simulink model "fcs_mpc"  (Simulink 9.0)
settings: Solver=VariableStepAuto  StartTime=0.0  StopTime=120  RelTol=1e-3
values from neighbouring files (symbols this model uses):
  Bf = 10000    [parameters.m]
  Bw = 1.7    [parameters.m]
  c = 2.1e-8    (= 2.1e-08)    [parameters.m]
  F_OmegaI = [-0.0162184150400002, -0.00631156082725452, -0.00162300350054704; 0.0162184150400002, 0.00631156082725452, 0.00162300350054704; -1.91252880199500e-16, 0.0704545731974788, 0; 1.91252880199500e-16, -0.0704545731974788, 0; 0.00203835199999989, 0.0823409037568373, 0.0338642741053293; -0.00203835199999989, -0.0823409037568373, -0.0338642741053293; -0.000739879228098683, -0.0271199969505346, 0.003148463 ...(+73 chars)    [parameters.m]
  F_OmegaO = [1, 0, 0; -1, 0, 0; 0, 1, 0; 0, -1, 0; 0, 0, 1; 0, 0, -1]    [parameters.m]
  g_OmegaI = [0.00133150970594632; 0.00133150970594632; 0.00320850126341322; 0.00320850126341322; 0.00334621106108639; 0.00334621106108639; 0.00174333401990860; 0.00174333401990860]    [parameters.m]
  g_OmegaO = [0.1; 0.1; 0.046; 0.046; 0.2; 0.2]    [parameters.m]
  Hc = 9    [parameters.m]
  Hp = 23    [parameters.m]
  initial_theta = deg2rad(9)    [parameters.m]
  initial_x = 0    [parameters.m]
  initial_y = 0.05    [parameters.m]
  J = 50    [parameters.m]
  Jw = 5    [parameters.m]
  K = 1    [parameters.m]
  Kp = 20    [parameters.m]
  L = Lr + Lf    (= 1.58)    [parameters.m]
  Lf = 0.79    [parameters.m]
  Lr = 0.79    [parameters.m]
  Lw = 0.54    [parameters.m]
  M = 250    [parameters.m]
  omega_f = 0.3253    [parameters.m]
  phi_max = 0.61    [parameters.m]
  R = 0.29    [parameters.m]
  r = 0.1    [parameters.m]
  speed_allow_direction = 0.1407    [parameters.m]
  speed_cost_coefficient = 5 / 3.6    (= 1.38888888889)    [parameters.m]
  step_time = 0.2    [parameters.m]
  trajectory = trajectory_straight    [parameters.m]
  varying_cost = false    [parameters.m]
libraries: simulink x6
settings Model: SuppressorTable=22 serialization::archive 11 0 6 0 0 0 11 0  Creator=root  LastModifiedBy=root
settings DataIOCC: SaveFormat=Dataset
settings OptimizationCC: LifeSpan=auto
settings DebuggingCC: UnderspecifiedInitializationDetection=Simplified  MergeDetectMultiDrivingBlocksExec=error  SFUnexpectedBacktrackingDiag=error  SFNoUnconditionalDefaultTransitionDiag=error  SFExecutionAtInitializationDiag=warning
settings HardwareCC: ProdBitPerPointer=64  ProdBitPerSizeT=64  ProdBitPerPtrDiffT=64  ProdLargestAtomicFloat=Float  ProdIntDivRoundTo=Zero  ProdEndianess=LittleEndian  ProdWordSize=64  ProdHWDeviceType=Intel->x86-64 (Windows64)
settings ModelReferenceCC: PropagateSignalLabelsOutOfModel=on
settings CodeAppCC: StateflowObjectComments=off
settings GRTTargetCC: TargetLangStandard=C99 (ISO)
settings ConfigComp: CovMetricSettings=dwe  CovHtmlReporting=off  CovSaveCumulativeToWorkspaceVar=off  CovSaveSingleToWorkspaceVar=off  CovExternalEMLEnable=on

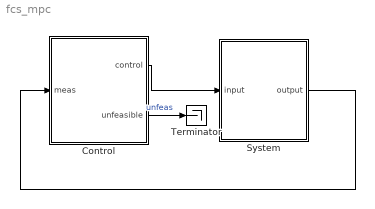
== system fcs_mpc ==
  Control : MATLAB Function  TreatAsAtomicUnit=on
  System : Subsystem
  Terminator : Terminator
  wires:
  Control/1(control) -> System/1(input)
  System/1(output) -> Control/1(meas)
  Control/2(unfeasible) -> Terminator/1  "unfeas"

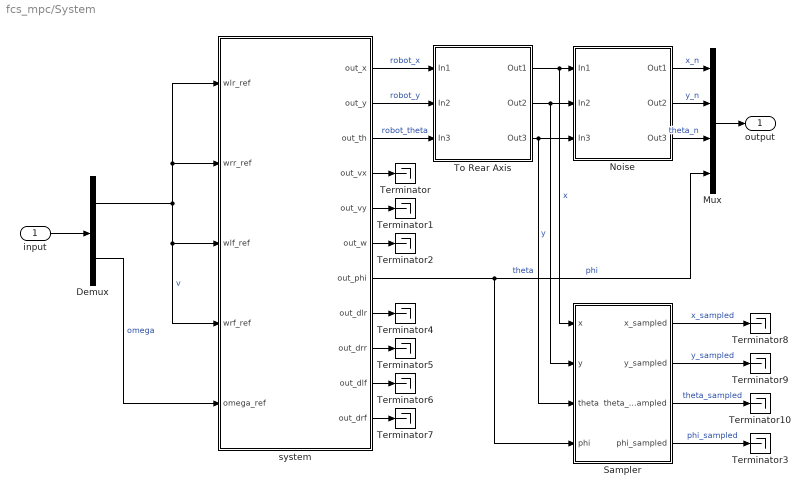
== system fcs_mpc/System ==
  input : Inport
  Demux : Demux  Outputs=2
  Mux : Mux
  Noise : Subsystem
  Sampler : MATLAB Function  TreatAsAtomicUnit=on
  Terminator{,1..10} (11 alike) : Terminator
  To Rear Axis : Subsystem
  system : Subsystem
  output : Outport
  wires:
  Demux/1 -> system/2(wrr_ref), system/1(wlr_ref), system/4(wrf_ref), system/3(wlf_ref)  "v"
  system/1(out_x) -> To Rear Axis/1(In1)  "robot_x"
  system/2(out_y) -> To Rear Axis/2(In2)  "robot_y"
  system/3(out_th) -> To Rear Axis/3(In3)  "robot_theta"
  Demux/2 -> system/5(omega_ref)  "omega"
  input/1 -> Demux/1
  Mux/1 -> output/1
  Noise/1(Out1) -> Mux/1  "x_n"
  Noise/2(Out2) -> Mux/2  "y_n"
  Noise/3(Out3) -> Mux/3  "theta_n"
  system/4(out_vx) -> Terminator/1
  system/5(out_vy) -> Terminator1/1
  system/6(out_w) -> Terminator2/1
  system/7(out_phi) -> Sampler/4(phi), Mux/4  "phi"
  system/8(out_dlr) -> Terminator4/1
  system/9(out_drr) -> Terminator5/1
  system/10(out_dlf) -> Terminator6/1
  system/11(out_drf) -> Terminator7/1
  Sampler/2(y_sampled) -> Terminator9/1  "y_sampled"
  Sampler/1(x_sampled) -> Terminator8/1  "x_sampled"
  To Rear Axis/2(Out2) -> Sampler/2(y), Noise/2(In2)  "y"
  To Rear Axis/1(Out1) -> Noise/1(In1), Sampler/1(x)  "x"
  To Rear Axis/3(Out3) -> Noise/3(In3), Sampler/3(theta)  "theta"
  Sampler/3(theta_sampled) -> Terminator10/1  "theta_sampled"
  Sampler/4(phi_sampled) -> Terminator3/1  "phi_sampled"

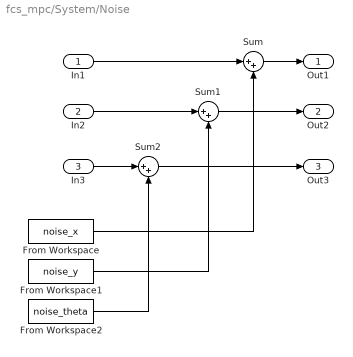
== system fcs_mpc/System/Noise ==
  In1 : Inport
  In2 : Inport  Port=2
  In3 : Inport  Port=3
  From Workspace : FromWorkspace  VariableName=noise_x  SampleTime=step_time  OutputAfterFinalValue=Holding final value
  From Workspace1 : FromWorkspace  VariableName=noise_y  SampleTime=step_time  OutputAfterFinalValue=Holding final value
  From Workspace2 : FromWorkspace  VariableName=noise_theta  SampleTime=step_time  OutputAfterFinalValue=Holding final value
  Sum : Sum  Inputs=|++
  Sum1 : Sum  Inputs=|++
  Sum2 : Sum  Inputs=|++
  Out1 : Outport
  Out2 : Outport  Port=2
  Out3 : Outport  Port=3
  wires:
  In3/1 -> Sum2/1
  From Workspace1/1 -> Sum1/2
  In1/1 -> Sum/1
  From Workspace2/1 -> Sum2/2
  From Workspace/1 -> Sum/2
  Sum2/1 -> Out3/1
  In2/1 -> Sum1/1
  Sum1/1 -> Out2/1
  Sum/1 -> Out1/1

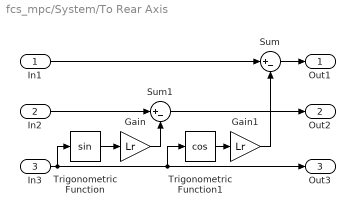
== system fcs_mpc/System/To Rear Axis ==
  In1 : Inport
  In2 : Inport  Port=2
  In3 : Inport  Port=3
  Gain : Gain  Gain=Lr
  Gain1 : Gain  Gain=Lr
  Sum : Sum  Inputs=|+-
  Sum1 : Sum  Inputs=|+-
  Trigonometric Function : Trigonometry
  Trigonometric Function1 : Trigonometry  Operator=cos
  Out1 : Outport
  Out2 : Outport  Port=2
  Out3 : Outport  Port=3
  wires:
  In1/1 -> Sum/1
  In2/1 -> Sum1/1
  Sum/1 -> Out1/1
  Sum1/1 -> Out2/1
  Trigonometric Function/1 -> Gain/1
  Gain/1 -> Sum1/2
  In3/1 -> Out3/1, Trigonometric Function1/1, Trigonometric Function/1
  Trigonometric Function1/1 -> Gain1/1
  Gain1/1 -> Sum/2

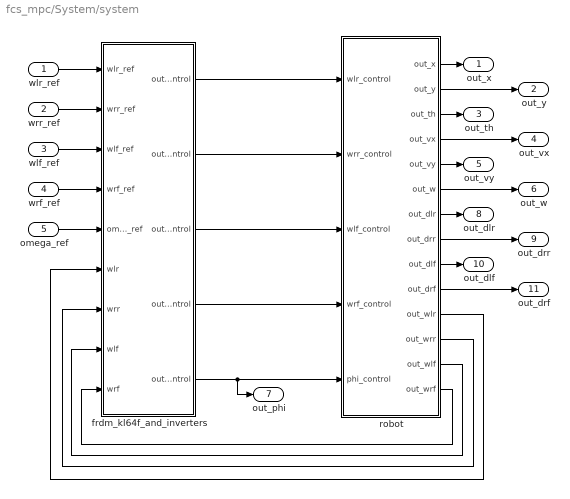
== system fcs_mpc/System/system ==
  wlr_ref : Inport
  wrr_ref : Inport  Port=2
  wlf_ref : Inport  Port=3
  wrf_ref : Inport  Port=4
  omega_ref : Inport  Port=5
  frdm_kl64f_and_inverters : Subsystem
  robot : Subsystem
  out_x : Outport
  out_y : Outport  Port=2
  out_th : Outport  Port=3
  out_vx : Outport  Port=4
  out_vy : Outport  Port=5
  out_w : Outport  Port=6
  out_phi : Outport  Port=7
  out_dlr : Outport  Port=8
  out_drr : Outport  Port=9
  out_dlf : Outport  Port=10
  out_drf : Outport  Port=11
  wires:
  wlr_ref/1 -> frdm_kl64f_and_inverters/1(wlr_ref)
  wrr_ref/1 -> frdm_kl64f_and_inverters/2(wrr_ref)
  wlf_ref/1 -> frdm_kl64f_and_inverters/3(wlf_ref)
  wrf_ref/1 -> frdm_kl64f_and_inverters/4(wrf_ref)
  omega_ref/1 -> frdm_kl64f_and_inverters/5(omega_ref)
  robot/11(out_wlr) -> frdm_kl64f_and_inverters/6(wlr)
  robot/12(out_wrr) -> frdm_kl64f_and_inverters/7(wrr)
  robot/13(out_wlf) -> frdm_kl64f_and_inverters/8(wlf)
  robot/14(out_wrf) -> frdm_kl64f_and_inverters/9(wrf)
  frdm_kl64f_and_inverters/1(outwlr_control) -> robot/1(wlr_control)
  frdm_kl64f_and_inverters/2(outwrr_control) -> robot/2(wrr_control)
  frdm_kl64f_and_inverters/3(outwlf_control) -> robot/3(wlf_control)
  frdm_kl64f_and_inverters/4(outwrf_control) -> robot/4(wrf_control)
  robot/1(out_x) -> out_x/1
  robot/2(out_y) -> out_y/1
  robot/3(out_th) -> out_th/1
  robot/5(out_vy) -> out_vy/1
  robot/7(out_dlr) -> out_dlr/1
  robot/9(out_dlf) -> out_dlf/1
  robot/10(out_drf) -> out_drf/1
  robot/8(out_drr) -> out_drr/1
  robot/6(out_w) -> out_w/1
  robot/4(out_vx) -> out_vx/1
  frdm_kl64f_and_inverters/5("outphi_control ") -> out_phi/1, robot/5(phi_control)

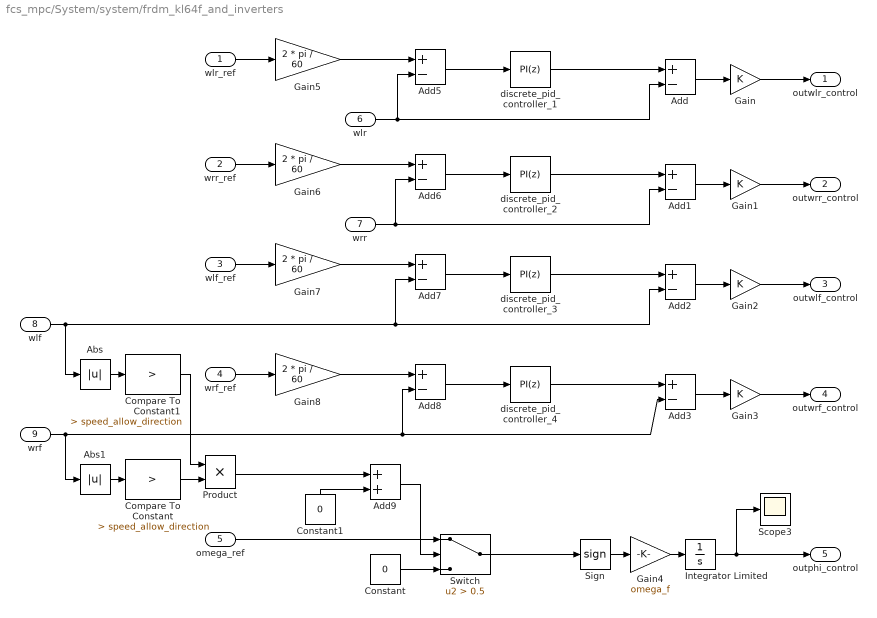
== system fcs_mpc/System/system/frdm_kl64f_and_inverters ==
  wlr_ref : Inport
  wrr_ref : Inport  Port=2
  wlf_ref : Inport  Port=3
  wrf_ref : Inport  Port=4
  omega_ref : Inport  Port=5
  wlr : Inport  Port=6
  wrr : Inport  Port=7
  wlf : Inport  Port=8
  wrf : Inport  Port=9
  Abs : Abs
  Abs1 : Abs
  Add{,1..3,5..8} (8 alike) : Sum  Inputs=+-
  Add9 : Sum
  Compare To Constant : simulink/Logic and Bit Operations/Compare To Constant  relop=>  const=speed_allow_direction  OutDataTypeStr=boolean
  Compare To Constant1 : simulink/Logic and Bit Operations/Compare To Constant  relop=>  const=speed_allow_direction  OutDataTypeStr=boolean
  Constant : Constant  Value=0
  Constant1 : Constant  Value=0
  Gain{,1..3} (4 alike) : Gain  Gain=K
  Gain4 : Gain  Gain=omega_f
  Gain{5..8} (4 alike) : Gain  Gain=2 * pi / 60
  Integrator Limited : Integrator  LimitOutput=on  UpperSaturationLimit=phi_max  LowerSaturationLimit=-phi_max
  Product : Product
  Scope3 : Scope
  Sign : Signum
  Switch : Switch  Criteria=u2 > Threshold  Threshold=0.5
  discrete_pid_controller_{1..4} (4 alike) : simulink/Continuous/PID Controller  Controller=PI  TimeDomain=Discrete-time  SampleTime=step_time  IntegratorMethod=Forward Euler  FilterMethod=Forward Euler  Form=Parallel  UseFilter=off  ControllerParametersSource=internal  P=Kp  I=Kp / Ti  D=0  N=100  InitialConditionSource=internal  InitialConditionForIntegrator=0  InitialConditionForFilter=0  ExternalReset=none  LimitOutput=off  UpperSaturationLimit=inf  LowerSaturationLimit=-inf  LinearizeAsGain=off  AntiWindupMode=none  Kb=1  TrackingMode=off  Kt=1  PParamMin=[]  PParamMax=[]  IParamMin=[]  IParamMax=[]  DParamMin=[]  DParamMax=[]  NParamMin=[]  NParamMax=[]  KbParamMin=[]  KbParamMax=[]  KtParamMin=[]  KtParamMax=[]  POutMin=[]  POutMax=[]  IOutMin=[]  IOutMax=[]  DOutMin=[]  DOutMax=[]  NOutMin=[]  NOutMax=[]  KbOutMin=[]  KbOutMax=[]  KtOutMin=[]  KtOutMax=[]  IntegratorOutMin=[]  IntegratorOutMax=[]  FilterOutMin=[]  FilterOutMax=[]  SumOutMin=[]  SumOutMax=[]  SumI1OutMin=[]  SumI1OutMax=[]  SumI2OutMin=[]  SumI2OutMax=[]  SumI3OutMin=[]  SumI3OutMax=[]  SumDOutMin=[]  SumDOutMax=[]  SaturationOutMin=[]  SaturationOutMax=[]  IntegratorContinuousStateAttributes=''  IntegratorStateMustResolveToSignalObject=off  IntegratorRTWStateStorageClass=Auto  FilterContinuousStateAttributes=''  FilterStateMustResolveToSignalObject=off  FilterRTWStateStorageClass=Auto  DifferentiatorICPrevScaledInput=0  DifferentiatorOutMin=[]  DifferentiatorOutMax=[]  InitialConditionSetting=State (most efficient)  FilterDiffOutCoefMin=[]  FilterDiffOutCoefMax=[]  SumDenOutMin=[]  SumDenOutMax=[]  SumNumOutMin=[]  SumNumOutMax=[]  ReciprocalOutMin=[]  ReciprocalOutMax=[]  DivideOutMin=[]  DivideOutMax=[]  TunerSelectOption=Transfer Function Based (PID Tuner App)
  outwlr_control : Outport
  outwrr_control : Outport  Port=2
  outwlf_control : Outport  Port=3
  outwrf_control : Outport  Port=4
  "outphi_control " : Outport  Port=5
  wires:
  Gain2/1 -> outwlf_control/1
  Gain4/1 -> Integrator Limited/1
  wrf/1 -> Abs1/1, Add8/2, Add3/2
  Sign/1 -> Gain4/1
  wrr/1 -> Add6/2, Add1/2
  Add7/1 -> discrete_pid_controller_3/1
  Add6/1 -> discrete_pid_controller_2/1
  Add3/1 -> Gain3/1
  wlr/1 -> Add5/2, Add/2
  Add/1 -> Gain/1
  Add1/1 -> Gain1/1
  wlf/1 -> Abs/1, Add7/2, Add2/2
  Add5/1 -> discrete_pid_controller_1/1
  discrete_pid_controller_4/1 -> Add3/1
  Add2/1 -> Gain2/1
  discrete_pid_controller_2/1 -> Add1/1
  Gain/1 -> outwlr_control/1
  Integrator Limited/1 -> Scope3/1, "outphi_control "/1
  discrete_pid_controller_3/1 -> Add2/1
  Add8/1 -> discrete_pid_controller_4/1
  Gain3/1 -> outwrf_control/1
  discrete_pid_controller_1/1 -> Add/1
  Gain1/1 -> outwrr_control/1
  wlr_ref/1 -> Gain5/1
  Gain5/1 -> Add5/1
  wrr_ref/1 -> Gain6/1
  Gain6/1 -> Add6/1
  wlf_ref/1 -> Gain7/1
  Gain7/1 -> Add7/1
  wrf_ref/1 -> Gain8/1
  Gain8/1 -> Add8/1
  Compare To Constant/1 -> Product/2
  Compare To Constant1/1 -> Product/1
  omega_ref/1 -> Switch/1
  Constant/1 -> Switch/3
  Abs/1 -> Compare To Constant1/1
  Abs1/1 -> Compare To Constant/1
  Constant1/1 -> Add9/2
  Product/1 -> Add9/1
  Switch/1 -> Sign/1
  Add9/1 -> Switch/2

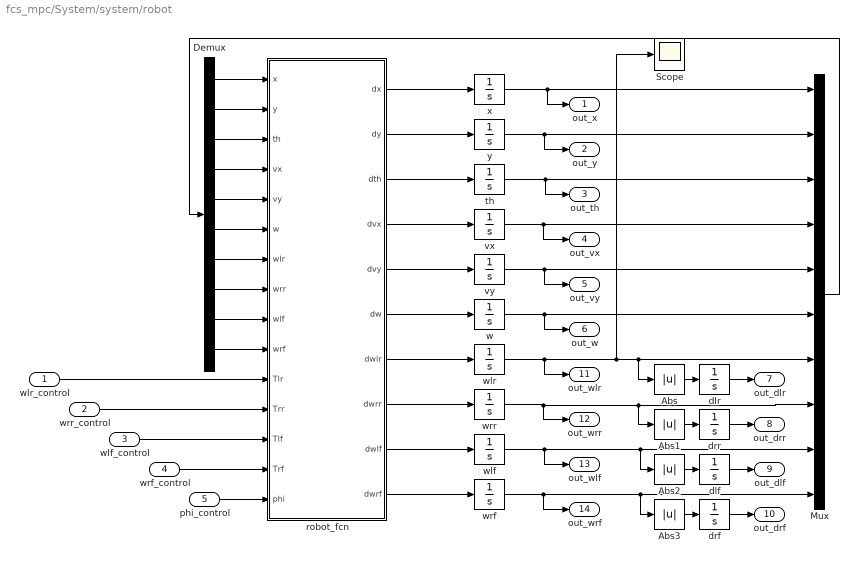
== system fcs_mpc/System/system/robot ==
  wlr_control : Inport
  wrr_control : Inport  Port=2
  wlf_control : Inport  Port=3
  wrf_control : Inport  Port=4
  phi_control : Inport  Port=5
  Abs{,1..3} (4 alike) : Abs
  Demux : Demux  Outputs=10
  Mux : Mux  Inputs=10
  Scope : Scope
  dlf : Integrator
  dlr : Integrator
  drf : Integrator
  drr : Integrator
  robot_fcn : MATLAB Function  TreatAsAtomicUnit=on
  th : Integrator  InitialCondition=initial_theta
  vx : Integrator
  vy : Integrator
  w : Integrator
  wlf : Integrator
  wlr : Integrator
  wrf : Integrator
  wrr : Integrator
  x : Integrator  InitialCondition=initial_x + Lr * cos(initial_theta)
  y : Integrator  InitialCondition=initial_y + Lr * sin(initial_theta)
  out_x : Outport
  out_y : Outport  Port=2
  out_th : Outport  Port=3
  out_vx : Outport  Port=4
  out_vy : Outport  Port=5
  out_w : Outport  Port=6
  out_dlr : Outport  Port=7
  out_drr : Outport  Port=8
  out_dlf : Outport  Port=9
  out_drf : Outport  Port=10
  out_wlr : Outport  Port=11
  out_wrr : Outport  Port=12
  out_wlf : Outport  Port=13
  out_wrf : Outport  Port=14
  wires:
  robot_fcn/1(dx) -> x/1
  drr/1 -> out_drr/1
  dlf/1 -> out_dlf/1
  Demux/8 -> robot_fcn/8(wrr)
  robot_fcn/6(dw) -> w/1
  th/1 -> out_th/1, Mux/3
  w/1 -> out_w/1, Mux/6
  wlf/1 -> out_wlf/1, Abs2/1, Mux/9
  y/1 -> out_y/1, Mux/2
  Mux/1 -> Demux/1
  robot_fcn/10(dwrf) -> wrf/1
  vy/1 -> Mux/5, out_vy/1
  vx/1 -> Mux/4, out_vx/1
  Demux/1 -> robot_fcn/1(x)
  robot_fcn/9(dwlf) -> wlf/1
  drf/1 -> out_drf/1
  Demux/5 -> robot_fcn/5(vy)
  robot_fcn/2(dy) -> y/1
  Demux/2 -> robot_fcn/2(y)
  robot_fcn/8(dwrr) -> wrr/1
  wrr_control/1 -> robot_fcn/12(Trr)
  wrf_control/1 -> robot_fcn/14(Trf)
  phi_control/1 -> robot_fcn/15(phi)
  Demux/9 -> robot_fcn/9(wlf)
  x/1 -> out_x/1, Mux/1
  robot_fcn/7(dwlr) -> wlr/1
  robot_fcn/5(dvy) -> vy/1
  Demux/6 -> robot_fcn/6(w)
  robot_fcn/4(dvx) -> vx/1
  Demux/10 -> robot_fcn/10(wrf)
  robot_fcn/3(dth) -> th/1
  wlf_control/1 -> robot_fcn/13(Tlf)
  Demux/7 -> robot_fcn/7(wlr)
  Demux/4 -> robot_fcn/4(vx)
  wrf/1 -> out_wrf/1, Abs3/1, Mux/10
  Demux/3 -> robot_fcn/3(th)
  wrr/1 -> out_wrr/1, Abs1/1, Mux/8
  dlr/1 -> out_dlr/1
  wlr_control/1 -> robot_fcn/11(Tlr)
  Abs/1 -> dlr/1
  Abs1/1 -> drr/1
  Abs2/1 -> dlf/1
  Abs3/1 -> drf/1
  wlr/1 -> out_wlr/1, Scope/1, Abs/1, Mux/7

== matlab function System/Sampler ==
  settings: updateMethod=DISCRETE  sampleTime=step_time/sampling_scale
  data: x input double; y input double; theta input double; x_sampled output double; y_sampled output double; theta_sampled output double; phi input double; phi_sampled output double
function [x_sampled,y_sampled, theta_sampled, phi_sampled] = fcn(x, y, theta, phi)
x_sampled = x;
y_sampled = y;
theta_sampled = theta;
phi_sampled = phi;

== matlab function System/system/robot/robot_fcn ==
  data: x input double; dx output double; y input double; th input double; vx input double; vy input double; w input double; wlr input double; wrr input double; wlf input double; wrf input double; Tlr input double; Trr input double; Tlf input double; Trf input double; phi input double; dy output double; dth output double; dvx output double; dvy output double; dw output double; dwlr output double; dwrr output double; dwlf output double; dwrf output double; Lr parameter double; Lf parameter double; Lw parameter double; R parameter double; M parameter double; J parameter double; Jw parameter double; Bw parameter double; Bf parameter double
function [dx, dy, dth, dvx, dvy, dw, dwlr, dwrr, dwlf, dwrf] = fcn(x, y, th, vx, vy, w, wlr, wrr, wlf, wrf, Tlr, Trr, Tlf, Trf, phi, Lr, Lf, Lw, R, M, J, Jw, Bw, Bf)

  vxlr = vx + (Lr * sin(th) - Lw * cos(th)) * w;
  vxrr = vx + (Lr * sin(th) + Lw * cos(th)) * w;
  vxlf = vx + (-Lf * sin(th) - Lw * cos(th)) * w;
  vxrf = vx + (-Lf * sin(th) + Lw * cos(th)) * w;
  vylr = vy + (-Lr * cos(th) - Lw * sin(th)) * w;
  vyrr = vy + (-Lr * cos(th) + Lw * sin(th)) * w;
  vylf = vy + (Lf * cos(th) - Lw * sin(th)) * w;
  vyrf = vy + (Lf * cos(th) + Lw * sin(th)) * w;

  Fxlr = Bf * (R * wlr * cos(th) - vxlr);
  Fylr = Bf * (R * wlr * sin(th) - vylr);
  Fxrr = Bf * (R * wrr * cos(th) - vxrr);
  Fyrr = Bf * (R * wrr * sin(th) - vyrr);
  Fxlf = Bf * (R * wlf * cos(th + phi) - vxlf);
  Fylf = Bf * (R * wlf * sin(th + phi) - vylf);
  Fxrf = Bf * (R * wrf * cos(th + phi) - vxrf);
  Fyrf = Bf * (R * wrf * sin(th + phi) - vyrf);

  taulr = Fxlr * sin(th) * Lr - Fxlr * cos(th) * Lw - Fylr * cos(th) * Lr - Fylr * sin(th) * Lw;
  taurr = Fxrr * sin(th) * Lr + Fxrr * cos(th) * Lw - Fyrr * cos(th) * Lr + Fyrr * sin(th) * Lw;
  taulf = -Fxlf * sin(th) * Lf - Fxlf * cos(th) * Lw + Fylf * cos(th) * Lf - Fylf * sin(th) * Lw;
  taurf = -Fxrf * sin(th) * Lf + Fxrf * cos(th) * Lw + Fyrf * cos(th) * Lf + Fylf * sin(th) * Lw;

  dx = vx;
  dy = vy;
  dth = w;
  dvx = (Fxlr + Fxrr + Fxlf + Fxrf) / M;
  dvy = (Fylr + Fyrr + Fylf + Fyrf) / M;
  dw = (taulr + taurr + taulf + taurf) / J;

  dwlr = (Tlr - R * Fxlr * cos(th) - R * Fylr * sin(th) - Bw * wlr) / Jw;
  dwrr = (Trr - R * Fxrr * cos(th) - R * Fyrr * sin(th) - Bw * wrr) / Jw;
  dwlf = (Tlf - R * Fxlf * cos(th + phi) - R * Fylf * sin(th + phi) - Bw * wlf) / Jw;
  dwrf = (Trf - R * Fxrf * cos(th + phi) - R * Fyrf * sin(th + phi) - Bw * wrf) / Jw;

== matlab function Control ==
  settings: updateMethod=DISCRETE  sampleTime=step_time
  data: meas input double; control output double; trajectory parameter double; Hp parameter double; Hc parameter double; step_time parameter double; R parameter double; phi_max parameter double; L parameter double; omega_f parameter double; F_OmegaI parameter double; g_OmegaI parameter double; F_OmegaO parameter double; g_OmegaO parameter double; r parameter double; c parameter double; unfeasible output double; varying_cost parameter double; speed_cost_coefficient parameter double
function [control,unfeasible] = fcn(meas, trajectory, Hp, Hc, step_time, R, phi_max, L, omega_f, F_OmegaI, g_OmegaI, F_OmegaO, g_OmegaO, r, c, varying_cost, speed_cost_coefficient)
    coder.extrinsic('FCS_MPC');
    control = zeros(2, 1);
    unfeasible = zeros(4, 1);
    [control, unfeasible] = FCS_MPC(meas, trajectory, Hp, Hc, step_time, R, phi_max, L, omega_f, F_OmegaI, g_OmegaI, F_OmegaO, g_OmegaO, r, c, varying_cost, speed_cost_coefficient);
